simulink model "AirtrimPioneer"  (R2018a)
settings: Solver=ode45  StartTime=0.0  StopTime=10.0  RelTol=1e-3  EnableMultiTasking=on
libraries: airlib x1
settings Model: Creator=SHETTYA1  LastModifiedBy=SHETTYA1
settings DataIOCC: ExternalInput=[0 1 0 0 0 0 0 0 0 0 6.7015280237240514e-017]  InitialState=[100;0.33384643595852526;0;0;0;0;0;0.33384643595852531;0;0;0;60]  LoadExternalInput=on  LoadInitialState=on  SaveFormat=Array  SignalLoggingSaveFormat=ModelDataLogs
settings OptimizationCC: BlockReduction=off  BooleanDataType=off
settings DebuggingCC: SaveWithParameterizedLinksMsg=none  UnderspecifiedInitializationDetection=Classic  MergeDetectMultiDrivingBlocksExec=none  SignalResolutionControl=TryResolveAllWithWarning  MultiTaskDSMMsg=warning  MultiTaskCondExecSysMsg=none
settings HardwareCC: TargetUnknown=on
settings ModelReferenceCC: PropagateSignalLabelsOutOfModel=off
settings GRTTargetCC: TargetLangStandard=C89/C90 (ANSI)  CombineOutputUpdateFcns=off  GRTInterface=on

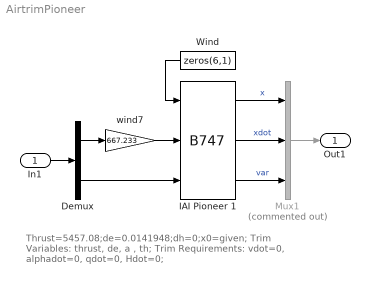
== system AirtrimPioneer ==
  note: Thrust=5457.08;de=0.0141948;dh=0;x0=given;
      | Trim Variables: thrust, de, a , th;
      | Trim Requirements: vdot=0, alphadot=0, qdot=0, Hdot=0;
  In1 : Inport
  " IAI Pioneer 1" : airlib/B747  GM1="[0.5486  5.1511  2.8261   47.2259  90.9483  111.4754   0  -6.6462  0   190.512]"  CD_wind="[0.060  0.430  0  0.0180  0]"  CL_wind="[0.385  4.78  8.05  0.401  0]"  Cm_body="[0.194  -2.12   -36.6   -1.76    0]"  CY_body="[0   -0.819    0     0    0.191    0]"  Cl_body="[0   -0.023   -0.450   0.265   -0.161  -0.00229]"  Cn_body="[0    0.109  -0.110  -0.200    0.0200  -0.0917]"  x0="[60 -0.0293682 0   0 0 0   0 -0.0293682 0   0 0 60]"
  Demux : Demux  Outputs=[6 4]
  Mux1 : Mux  Commented=on  Inputs=[12 12 12]
  Wind : Constant  Value=zeros(6,1)
  wind7 : Gain  Gain=667.233  SaturateOnIntegerOverflow=on  OutDataTypeStr=Inherit: Same as input  ParamDataTypeStr=Inherit: Same as input
  Out1 : Outport
  wires:
  Demux/1 -> wind7/1
  In1/1 -> Demux/1
  Mux1/1 -> Out1/1
  Wind/1 -> " IAI Pioneer 1"/1
  wind7/1 -> " IAI Pioneer 1"/2
  Demux/2 -> " IAI Pioneer 1"/3
  " IAI Pioneer 1"/1 -> Mux1/1  "x"
  " IAI Pioneer 1"/2 -> Mux1/2  "xdot"
  " IAI Pioneer 1"/3 -> Mux1/3  "var"
